simulink library "lib_fuel_converter3"  (Simulink 4.1.1)
values from neighbouring files (symbols this model uses):
  logFlag = 1    [advSACompMaskInit.m]    (also in advSACompMaskInitR13.m)
undefined symbols (not defined in the file or in its folder): air_cp, amb_tmp, cyc_mph, ex_gas_cp, fc_acc_mass, fc_base_mass, fc_c2i_th_cond, fc_c_init_tmp, fc_cl2h_eff, fc_CO2_to_FUELgps, fc_cold, fc_cold_tmp, fc_cp, fc_ct_trq, fc_emisv, fc_ext_sarea, fc_fuel_den, fc_fuel_lhv, fc_h2x_th_cond, fc_h_air_flow, fc_h_cp, fc_h_init_tmp, fc_hood_emisv, fc_hood_sarea, fc_i2x_th_cond, fc_i_init_tmp, fc_inertia, fc_map_spd, fc_map_trq, fc_max_trq, fc_nn_model_name, fc_pwr_scale, fc_spd_scale, fc_trq_scale, fc_tstat, fc_x_init_tmp, fd_ratio, gb_num_init, gb_ratio, generalName, pow, vc_idle_bool, vc_idle_spd, vc_key_on, veh_glider_mass, wh_radius
libraries: lib_fuel_converter3 x4, lib_etc x4, lib_fuel_converter x2, lib_fuel_converter2 x1
(part 9 of 9)

== system lib_fuel_converter3/fuel converter <fc> no fuel at negative torque/IC Engine Model  &  Interface/ic engine model/fuel use and EO emis no fuel used at negative torque/fc temp correct/fc temp correct Variable Correction Factors (Map Based)/NOx factor cold-to-hot ==
  x0 : Inport  Port=1  LatchInput=off
  y0 : Inport  Port=2  LatchInput=off
  Mux : Mux  Inputs=2
      settings: DisplayOption=none
  S-function : S-Function  FunctionName=sftable2  Parameters=xindex, yindex, table  PortCounts=[]  SFunctionModules=''
  table out : Outport  Port=1  InitialOutput=0
  wires:
  y0/1 -> Mux/2
  S-function/1 -> table out/1
  x0/1 -> Mux/1
  Mux/1 -> S-function/1

== system lib_fuel_converter3/fuel converter <fc> no fuel at negative torque/IC Engine Model  &  Interface/ic engine model/fuel use and EO emis no fuel used at negative torque/fc temp correct/fc temp correct Variable Correction Factors (Map Based)/PM factor cold-to-hot ==
  x0 : Inport  Port=1  LatchInput=off
  y0 : Inport  Port=2  LatchInput=off
  Mux : Mux  Inputs=2
      settings: DisplayOption=none
  S-function : S-Function  FunctionName=sftable2  Parameters=xindex, yindex, table  PortCounts=[]  SFunctionModules=''
  table out : Outport  Port=1  InitialOutput=0
  wires:
  y0/1 -> Mux/2
  S-function/1 -> table out/1
  x0/1 -> Mux/1
  Mux/1 -> S-function/1

== system lib_fuel_converter3/fuel converter <fc> no fuel at negative torque/IC Engine Model  &  Interface/ic engine model/fuel use and EO emis no fuel used at negative torque/fc temp correct/fc temp correct Variable Correction Factors (Map Based)/fuel factor cold-to-hot ==
  x0 : Inport  Port=1  LatchInput=off
  y0 : Inport  Port=2  LatchInput=off
  Mux : Mux  Inputs=2
      settings: DisplayOption=none
  S-function : S-Function  FunctionName=sftable2  Parameters=xindex, yindex, table  PortCounts=[]  SFunctionModules=''
  table out : Outport  Port=1  InitialOutput=0
  wires:
  y0/1 -> Mux/2
  S-function/1 -> table out/1
  x0/1 -> Mux/1
  Mux/1 -> S-function/1
